simulink model "Fig05"  (R2023b)
settings: Solver=ode1  StartTime=0.0  StopTime=600  FixedStep=1  RelTol=1e-3
settings Model: Creator=orlandojorquera  LastModifiedBy=evogel

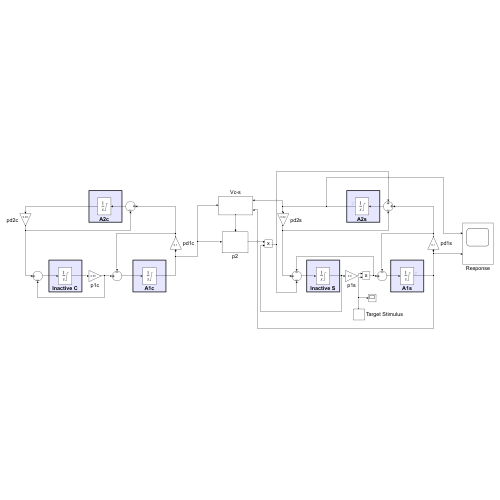
[thumbnail: Simulink's stored preview of the top-level diagram]
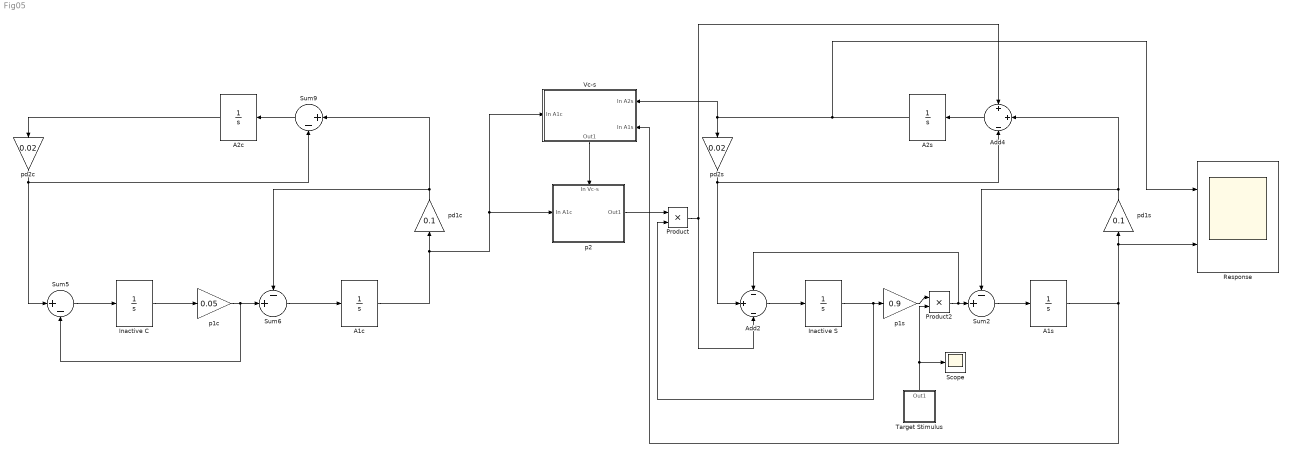
== system Fig05 ==
  A1c : Integrator  LimitOutput=on  LowerSaturationLimit=0
  A1s : Integrator  LimitOutput=on  LowerSaturationLimit=0
  A2c : Integrator  LimitOutput=on  LowerSaturationLimit=0
  A2s : Integrator  LimitOutput=on  LowerSaturationLimit=0
  Add2 : Sum  Inputs=-|+|-
  Add4 : Sum  Inputs=+|+|-
  Inactive C : Integrator  InitialCondition=1  LimitOutput=on  LowerSaturationLimit=0
  Inactive S : Integrator  InitialCondition=1  LimitOutput=on  LowerSaturationLimit=0
  Product : Product
  Product2 : Product
  Response : Scope  NumInputPorts=2
  Scope : Scope
  Sum2 : Sum  Inputs=-+|
  Sum5 : Sum  Inputs=|+-
  Sum6 : Sum  Inputs=-+|
  Sum9 : Sum  Inputs=|+-
  Target Stimulus : Subsystem
  Vc-s : Subsystem
      settings: PortSchema="{\"entries\":[{\"content\":{\"sides\":[{\"content\":{\"connectorIds\":[\"In1\"]},\"type\":\"ConnectorPlacement.EquallySpacedRectSide\",\"uuid\":\"b09f05bd-5603-47fe-a5ad-d7d6b3dc0c8e\"},{\"content\":{\"connectorIds\":[\"In2\",\"In3\"],\"side\":\"RIGHT\"},\"type\":\"ConnectorPlacement.EquallySpacedRectSide\",\"uuid\":\"d47795f3-6d8c-4c23-a554-34b772022c1b\"},{\"content\":{\"side\":\"TOP\"},\"type\":\"ConnectorPlacement.EquallySpacedRectSide\",\"uuid\":\"e48eddfd-d331-425c-b357-ebbea553df38\"},{\"content\":{\"connectorIds\":[\"Out1\"],\"side\":\"BOTTOM\"},\"type\":\"ConnectorPlacement.EquallySpacedRectSide\",\"uuid\":\"833a9385-f8e7-4f69-9c09-473a519a1ef8\"}]},\"type\":\"ConnectorPlacement.EquallySpacedConnector\",\"uuid\":\"43dd1673-4710-4827-90f7-71f5e88827f7\"}],\"packageUris\":[\"http://schema.mathworks.com/mf0/Connector/R2020b\"],\"version\":\"1.0\"}"
  p1c : Gain  Gain=0.05
  p1s : Gain  Gain=0.9
  p2 : Subsystem
      settings: PortSchema="{\"entries\":[{\"content\":{\"sides\":[{\"content\":{\"connectorIds\":[\"In1\"]},\"type\":\"ConnectorPlacement.EquallySpacedRectSide\",\"uuid\":\"e5de33b1-e289-4f06-b16e-f6995d6ff18d\"},{\"content\":{\"connectorIds\":[\"Out1\"],\"side\":\"RIGHT\"},\"type\":\"ConnectorPlacement.EquallySpacedRectSide\",\"uuid\":\"bf82b542-ee2f-4a07-ac72-0e3e2437644b\"},{\"content\":{\"connectorIds\":[\"In2\"],\"side\":\"TOP\"},\"type\":\"ConnectorPlacement.EquallySpacedRectSide\",\"uuid\":\"dbd75b9a-fc8b-4088-9d34-f07ad0492047\"}]},\"type\":\"ConnectorPlacement.EquallySpacedConnector\",\"uuid\":\"24fb73df-5fe4-4caa-a2a9-0eaf37dbdd75\"}],\"packageUris\":[\"http://schema.mathworks.com/mf0/Connector/R2020b\"],\"version\":\"1.0\"}"
  pd1c : Gain  Gain=0.1
  pd1s : Gain  Gain=0.1
  pd2c : Gain  Gain=0.02
  pd2s : Gain  Gain=0.02
  wires:
  Inactive C/1 -> p1c/1
  Sum5/1 -> Inactive C/1
  p1c/1 -> Sum6/2, Sum5/2
  pd1c/1 -> Sum9/1, Sum6/1
  Sum6/1 -> A1c/1
  A1c/1 -> Vc-s/1(In A1c), p2/1(In A1c), pd1c/1
  Sum9/1 -> A2c/1
  A2c/1 -> pd2c/1
  pd2c/1 -> Sum5/1, Sum9/2
  Vc-s/1(Out1) -> p2/2(In Vc-s)
  pd2s/1 -> Add4/3, Add2/2
  A2s/1 -> Response/1, pd2s/1, Vc-s/2(In A2s)
  Add4/1 -> A2s/1
  A1s/1 -> Response/2, pd1s/1, Vc-s/3(In A1s)
  Sum2/1 -> A1s/1
  pd1s/1 -> Add4/2, Sum2/1
  Add2/1 -> Inactive S/1
  Inactive S/1 -> Product/2, p1s/1
  Product2/1 -> Add2/1, Sum2/2
  p1s/1 -> Product2/1
  Target Stimulus/1(Out1) -> Scope/1, Product2/2
  p2/1(Out1) -> Product/1
  Product/1 -> Add2/3, Add4/1

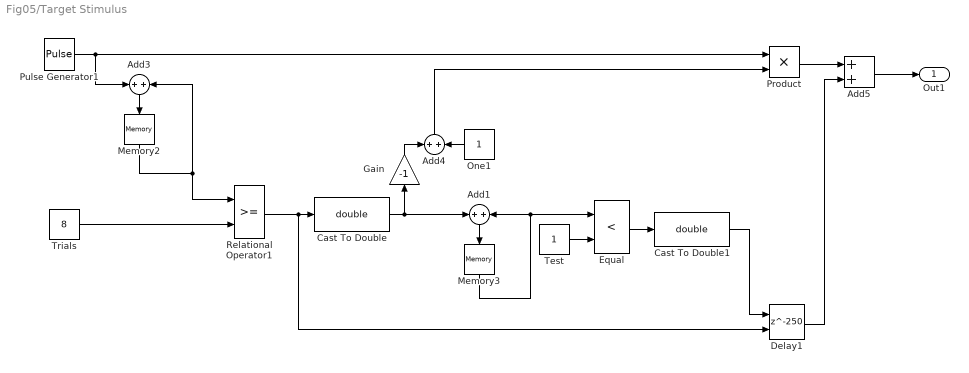
== system Fig05/Target Stimulus ==
  Add{1,3..5} (4 alike) : Sum
  Cast To Double : DataTypeConversion  OutDataTypeStr=double  SaturateOnIntegerOverflow=off  RndMeth=Floor
  Cast To Double1 : DataTypeConversion  OutDataTypeStr=double  SaturateOnIntegerOverflow=off  RndMeth=Floor
  Delay1 : Delay  DelayLength=250  ShowEnablePort=on
      settings: InputPortMap=u0,e6
  Equal : RelationalOperator  Operator=<  OutDataTypeStr=boolean  RndMeth=Simplest  InputSameDT=off
  Gain : Gain  Gain=-1
  Memory2 : Memory
  Memory3 : Memory
  One1 : Constant  OutDataTypeStr=Inherit: Inherit via back propagation
  Product : Product
  Pulse Generator1 : DiscretePulseGenerator  Period=10  PhaseDelay=180
  Relational Operator1 : RelationalOperator  OutDataTypeStr=boolean  RndMeth=Simplest  InputSameDT=off
  Test : Constant  OutDataTypeStr=Inherit: Inherit via back propagation
  Trials : Constant  Value=8
  Out1 : Outport
  wires:
  Pulse Generator1/1 -> Add3/1, Product/1
  Add3/1 -> Memory2/1
  Memory2/1 -> Relational Operator1/1, Add3/2
  Trials/1 -> Relational Operator1/2
  Relational Operator1/1 -> Delay1/2, Cast To Double/1
  Cast To Double/1 -> Gain/1, Add1/1
  Add1/1 -> Memory3/1
  Memory3/1 -> Add1/2, Equal/1
  Test/1 -> Equal/2
  Equal/1 -> Cast To Double1/1
  Gain/1 -> Add4/1
  One1/1 -> Add4/2
  Add4/1 -> Product/2
  Cast To Double1/1 -> Delay1/1
  Product/1 -> Add5/1
  Delay1/1 -> Add5/2
  Add5/1 -> Out1/1

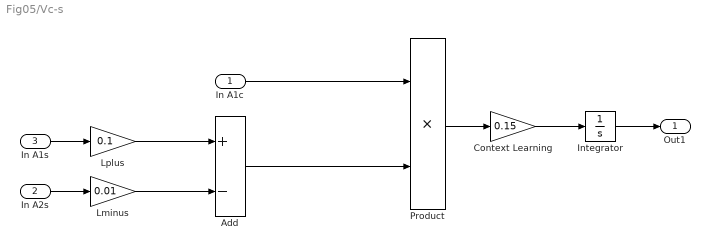
== system Fig05/Vc-s ==
  In A1c : Inport
  In A2s : Inport  Port=2
  In A1s : Inport  Port=3
  Add : Sum  Inputs=+-
  Context Learning : Gain  Gain=0.15
  Integrator : Integrator  LimitOutput=on  LowerSaturationLimit=0
  Lminus : Gain  Gain=0.01
  Lplus : Gain  Gain=0.1
  Product : Product
  Out1 : Outport
  wires:
  In A1s/1 -> Lplus/1
  In A2s/1 -> Lminus/1
  In A1c/1 -> Product/1
  Product/1 -> Context Learning/1
  Context Learning/1 -> Integrator/1
  Add/1 -> Product/2
  Lplus/1 -> Add/1
  Lminus/1 -> Add/2
  Integrator/1 -> Out1/1

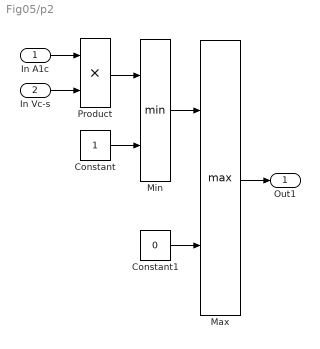
== system Fig05/p2 ==
  In A1c : Inport
  In Vc-s : Inport  Port=2
  Constant : Constant
  Constant1 : Constant  Value=0
  Max : MinMax  Function=max  Inputs=2
  Min : MinMax  Inputs=2
  Product : Product
  Out1 : Outport
  wires:
  In Vc-s/1 -> Product/2
  In A1c/1 -> Product/1
  Product/1 -> Min/1
  Constant/1 -> Min/2
  Min/1 -> Max/1
  Constant1/1 -> Max/2
  Max/1 -> Out1/1
